simulink model "ins_ideal"  (R2026a)
settings: configuration reference "standardSILConfiguraitonParams" (kept outside this file)
undefined symbols (not defined in the file or in its folder): stepSize_s
libraries: aerolibnav x1, simulink x1
settings Model: Creator=GTAR  LastModifiedBy=Edison Altamirano
settings ConfigSetRef: SourceName=standardSILConfiguraitonParams  SourceLocation=Base Workspace

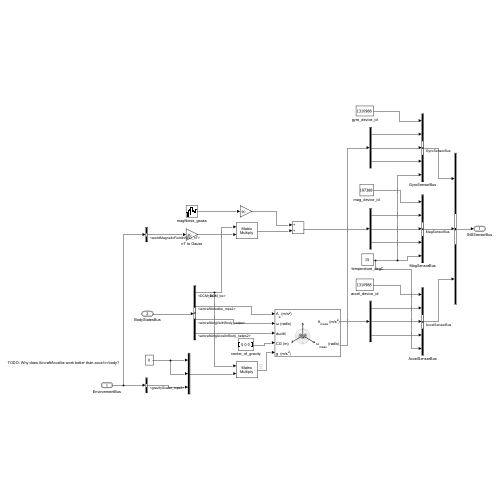
[thumbnail: Simulink's stored preview of the top-level diagram]
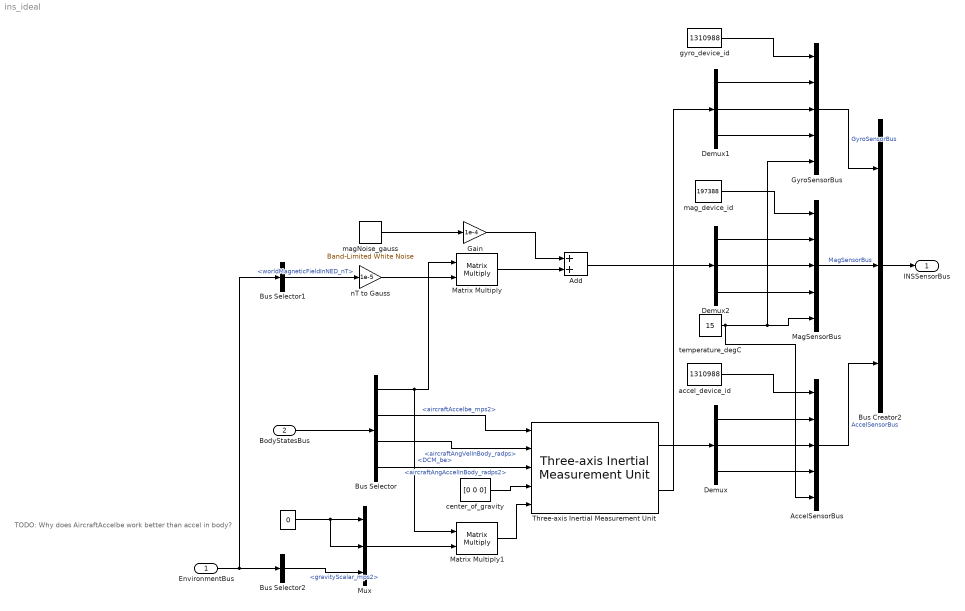
== system ins_ideal ==
  note: TODO: Why does AircraftAccelbe work better than accel in body?
  EnvironmentBus : Inport  OutDataTypeStr=Bus: EnvironmentBus
  BodyStatesBus : Inport  Port=2  OutDataTypeStr=Bus: BodyStateBus
  " " : Constant  Value=0  VectorParams1D=off  OutDataTypeStr=double
  AccelSensorBus : BusCreator  Inputs=5  OutDataTypeStr=Bus: AccelSensorBus
      settings: InheritFromInputs=off
  Add : Sum
  Bus Selector : BusSelector  OutputSignals=DCM_be,aircraftAccelbe_mps2,aircraftAngVelInBody_radps,aircraftAngAccelInBody_radps2
  Bus Selector1 : BusSelector  OutputSignals=EarthEnvironment.worldMagneticFieldInNED_nT
  Bus Selector2 : BusSelector  OutputSignals=EarthEnvironment.gravityScalar_mps2
  Bus Creator2 : BusCreator  Inputs=3  OutDataTypeStr=Bus: INSSensorBus
      settings: InheritFromInputs=off
  Demux : Demux  Outputs=3
  Demux1 : Demux  Outputs=3
  Demux2 : Demux  Outputs=3
  Gain : Gain  Gain=1e-4
  GyroSensorBus : BusCreator  Inputs=5  OutDataTypeStr=Bus: GyroSensorBus
      settings: InheritFromInputs=off
  MagSensorBus : BusCreator  Inputs=5  OutDataTypeStr=Bus: MagSensorBus
      settings: InheritFromInputs=off
  Matrix Multiply : Product  Multiplication=Matrix(*)
  Matrix Multiply1 : Product  Multiplication=Matrix(*)
  Mux : Mux  Inputs=3
  Three-axis Inertial Measurement Unit : aerolibnav/Three-axis Inertial Measurement Unit  units=Metric (MKS)  imu=[0 0 0]  i_Ts=stepSize_s  dtype_a=off  w_a=parameters.accel.naturalFrequency_radps  z_a=parameters.accel.dampingRatio_nd  a_sf_cc=eye(3)  a_bias=[0 0 0]  a_sat=[-1e6 -1e6 -1e6 1e6 1e6 1e6]  dtype_g=off  w_g=parameters.gyro.naturalFrequency_radps  z_g=parameters.gyro.dampingRatio_nd  g_sf_cc=eye(3)  g_bias=[0 0 0]  g_sens=[0 0 0]  g_sat=[-1e6 -1e6 -1e6 1e6 1e6 1e6]  i_rand=off  i_seeds=[23093 23094 23095 23096 23097 23098]  i_pow=zeros(1,6)
  accel_device_id : Constant  Value=1310988  OutDataTypeStr=double  LockScale=on
  center_of_gravity : Constant  Value=[0 0 0]  VectorParams1D=off  OutDataTypeStr=double
  gyro_device_id : Constant  Value=1310988  OutDataTypeStr=double  LockScale=on
  magNoise_gauss : simulink/Sources/Band-Limited White Noise  Cov=parameters.mag.noisePower_gauss  Ts=stepSize_s  seed=[23341 2873 29]
  mag_device_id : Constant  Value=197388  OutDataTypeStr=double  LockScale=on
  nT to Gauss : Gain  Gain=1e-5
  temperature_degC : Constant  Value=15  OutDataTypeStr=Inherit: Inherit via back propagation
  INSSensorBus : Outport  OutDataTypeStr=Bus: INSSensorBus
  wires:
  EnvironmentBus/1 -> Bus Selector2/1, Bus Selector1/1
  Bus Selector1/1 -> nT to Gauss/1  "<worldMagneticFieldInNED_nT>"
  Bus Selector/1 -> Matrix Multiply/1, Matrix Multiply1/1  "<DCM_be>"
  BodyStatesBus/1 -> Bus Selector/1
  temperature_degC/1 -> MagSensorBus/5, GyroSensorBus/5, AccelSensorBus/5
  Bus Selector2/1 -> Mux/3  "<gravityScalar_mps2>"
  " "/1 -> Mux/2, Mux/1
  Demux/3 -> AccelSensorBus/4
  magNoise_gauss/1 -> Gain/1
  nT to Gauss/1 -> Matrix Multiply/2
  Bus Selector/3 -> Three-axis Inertial Measurement Unit/2  "<aircraftAngVelInBody_radps>"
  Bus Selector/2 -> Three-axis Inertial Measurement Unit/1  "<aircraftAccelbe_mps2>"
  Bus Selector/4 -> Three-axis Inertial Measurement Unit/3  "<aircraftAngAccelInBody_radps2>"
  Mux/1 -> Matrix Multiply1/2
  Gain/1 -> Add/1
  Matrix Multiply/1 -> Add/2
  Bus Creator2/1 -> INSSensorBus/1
  center_of_gravity/1 -> Three-axis Inertial Measurement Unit/4
  Matrix Multiply1/1 -> Three-axis Inertial Measurement Unit/5
  accel_device_id/1 -> AccelSensorBus/1
  Add/1 -> Demux2/1
  Three-axis Inertial Measurement Unit/1 -> Demux/1
  Three-axis Inertial Measurement Unit/2 -> Demux1/1
  Demux/2 -> AccelSensorBus/3
  Demux/1 -> AccelSensorBus/2
  gyro_device_id/1 -> GyroSensorBus/1
  mag_device_id/1 -> MagSensorBus/1
  Demux1/1 -> GyroSensorBus/2
  Demux1/3 -> GyroSensorBus/4
  Demux1/2 -> GyroSensorBus/3
  Demux2/2 -> MagSensorBus/3
  Demux2/1 -> MagSensorBus/2
  Demux2/3 -> MagSensorBus/4
  GyroSensorBus/1 -> Bus Creator2/1  "GyroSensorBus"
  MagSensorBus/1 -> Bus Creator2/2  "MagSensorBus"
  AccelSensorBus/1 -> Bus Creator2/3  "AccelSensorBus"
